simulink model "Adaptive_control_CSAD_model"  (R2017a)
settings: Solver=ode4  StartTime=0.0  StopTime=t_sim  FixedStep=0.01  RelTol=1e-3
values from neighbouring files (symbols this model uses):
  controller = 1    [Run4corner.m]
  eta_initial = [5; -1; 0]    [Run4corner.m]    (also in Simulation_plot.m = [-4; -2; 0.6*pi])
  gamma = 1.5    [Run4corner.m]
  mrs_select = 0    [Run4corner.m]
  nu_initial = [0; 0; 0]    [Run4corner.m]    (also in Simulation_plot.m)
  rho = 0.8    [Run4corner.m]
  sigma = 2    [Run4corner.m]
undefined symbols (not defined in the file or in its folder): fdesignblkfcn, gcbh
libraries: simulink x4, dsparch4 x1
(part 1 of 2)
settings Model: Creator=torees  LastModifiedBy=torees

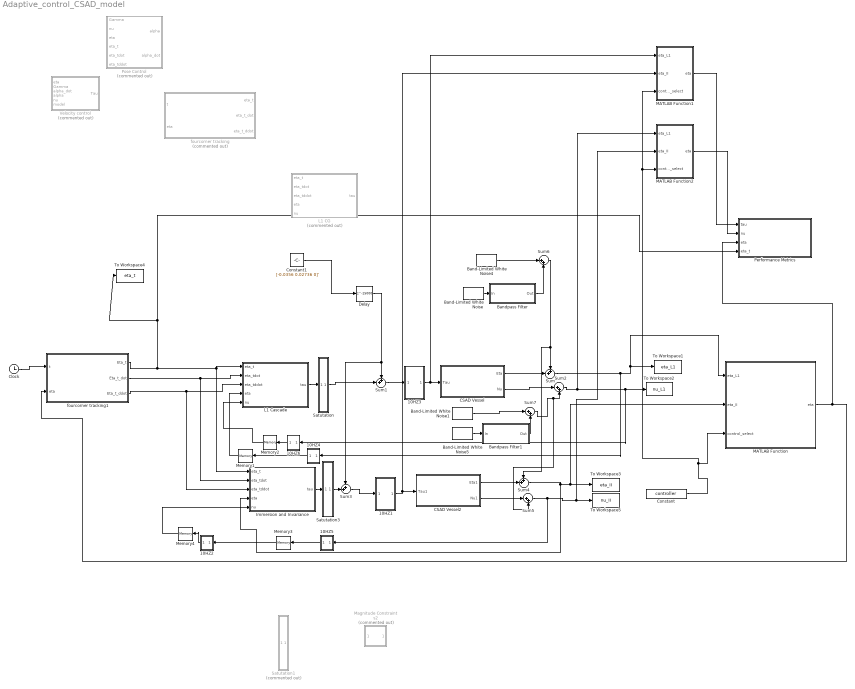
== system Adaptive_control_CSAD_model ==
  10HZ1 : Subsystem
  10HZ2 : Subsystem
  10HZ3 : Subsystem
  10HZ4 : Subsystem
  10HZ5 : Subsystem
  10HZ6 : Subsystem
  Band-Limited White Noise : simulink/Sources/Band-Limited White Noise  Cov=posnoise  Ts=0.01  seed=[233451]
  Band-Limited White Noise1 : simulink/Sources/Band-Limited White Noise  Cov=velnoise2  Ts=0.01  seed=[233451]
  Band-Limited White Noise4 : simulink/Sources/Band-Limited White Noise  Cov=posnoise2  Ts=0.01  seed=[233451]
  Band-Limited White Noise5 : simulink/Sources/Band-Limited White Noise  Cov=velnoise  Ts=0.01  seed=[233451]
  Bandpass Filter : Subsystem  DialogController=fdesignblkfcn  InitFcn=fdesignblkfcn(gcbh, {'InitFcn'});  mask(Bandpass Filter){}
      mask help: Design a bandpass filter
      settings: CopyFcn=fdesignblkfcn(gcbh, {'CopyFcn'});
      mask Help: helpview(mapfilelocation('dsp'), 'dspbandpassfilter');
      mask Display: disp('Bandpass');
  Bandpass Filter1 : Subsystem  DialogController=fdesignblkfcn  InitFcn=fdesignblkfcn(gcbh, {'InitFcn'});  mask(Bandpass Filter){}
      mask help: Design a bandpass filter
      settings: CopyFcn=fdesignblkfcn(gcbh, {'CopyFcn'});
      mask Help: helpview(mapfilelocation('dsp'), 'dspbandpassfilter');
      mask Display: disp('Bandpass');
  CSAD Vessel : Subsystem
  CSAD Vessel2 : Subsystem
  Clock : Clock
  Constant : Constant  Value=controller
  Constant1 : Constant  Value=[-0.0356 0.02736 0]'
  Delay : Delay  DelayLength=15000  InitialCondition=0
  Immersion and Invariance : Subsystem
  L1 CG : Subsystem  Commented=on
  L1 Cascade : Subsystem
  MATLAB Function : MATLAB Function  TreatAsAtomicUnit=on
  MATLAB Function1 : MATLAB Function  TreatAsAtomicUnit=on
  MATLAB Function2 : MATLAB Function  TreatAsAtomicUnit=on
  Magnitude Constraints2 : MATLAB Function  Commented=on  TreatAsAtomicUnit=on
  Memory{1..4} (4 alike) : Memory  X0=[ 0 0 0]'
  "Performance Metrics " : Subsystem
  Pose Control : Subsystem  Commented=on
  Satutation : Subsystem
  Satutation1 : Subsystem  Commented=on
  Satutation3 : Subsystem
  Sum{,1,3..4} (4 alike) : Sum  Inputs=++|
  Sum{2,5..7} (4 alike) : Sum  Inputs=|++
  To Workspace1 : ToWorkspace  VariableName=eta_L1  SampleTime=-1
  To Workspace2 : ToWorkspace  VariableName=nu_L1  SampleTime=-1
  To Workspace3 : ToWorkspace  VariableName=eta_II  SampleTime=-1
  To Workspace4 : ToWorkspace  VariableName=eta_t  SampleTime=-1
  To Workspace5 : ToWorkspace  VariableName=nu_II  SampleTime=-1
  Velocity control : Subsystem  Commented=on
  fourcorner tracking : Subsystem  Commented=on
  fourcorner tracking1 : MATLAB Function  TreatAsAtomicUnit=on
  wires:
  Clock/1 -> fourcorner tracking1/1(t)
  Constant/1 -> MATLAB Function2/3(control_select), MATLAB Function1/3(control_select), MATLAB Function/3(control_select)
  MATLAB Function/1(eta) -> "Performance Metrics "/3(eta), fourcorner tracking1/2(eta)
  CSAD Vessel/1(Eta) -> Sum/2
  fourcorner tracking1/2(Eta_t_dot) -> L1 Cascade/2(eta_tdot), Immersion and Invariance/2(eta_tdot)
  fourcorner tracking1/3(Eta_t_ddot) -> L1 Cascade/3(eta_tddot), Immersion and Invariance/3(eta_tddot)
  Band-Limited White Noise/1 -> Bandpass Filter/1(In)
  10HZ3/1(Out1) -> MATLAB Function1/1(eta_L1), CSAD Vessel/1(Tau)
  Sum/1 -> 10HZ4/1(In1), MATLAB Function/1(eta_L1), To Workspace1/1
  fourcorner tracking1/1(Eta_t) -> To Workspace4/1, "Performance Metrics "/4(eta_t), L1 Cascade/1(eta_t), Immersion and Invariance/1(eta_t)
  L1 Cascade/1(tau) -> Satutation/1(In1)
  Sum1/1 -> 10HZ3/1(In1)
  CSAD Vessel/2(Nu) -> Sum2/1
  Sum7/1 -> Sum5/2, Sum2/2
  Sum2/1 -> MATLAB Function2/1(eta_L1), 10HZ6/1(In1), To Workspace2/1
  Delay/1 -> Sum3/1, Sum1/1
  Immersion and Invariance/1(tau) -> Satutation3/1(In1)
  Sum3/1 -> 10HZ1/1(In1)
  CSAD Vessel2/1(Eta1) -> Sum4/2
  CSAD Vessel2/2(Nu1) -> Sum5/1
  Sum5/1 -> 10HZ5/1(In1), MATLAB Function2/2(eta_II), To Workspace5/1
  Sum4/1 -> Immersion and Invariance/4(eta), MATLAB Function/2(eta_II), To Workspace3/1
  10HZ1/1(Out1) -> CSAD Vessel2/1(Tau1), MATLAB Function1/2(eta_II)
  MATLAB Function1/1(eta) -> "Performance Metrics "/1(tau)
  MATLAB Function2/1(eta) -> "Performance Metrics "/2(nu)
  Satutation/1(Out1) -> Sum1/2
  Satutation3/1(Out1) -> Sum3/2
  Bandpass Filter/1(Out) -> Sum6/2
  Sum6/1 -> Sum4/1, Sum/1
  Band-Limited White Noise4/1 -> Sum6/1
  Bandpass Filter1/1(Out) -> Sum7/2
  Band-Limited White Noise5/1 -> Bandpass Filter1/1(In)
  Band-Limited White Noise1/1 -> Sum7/1
  Constant1/1 -> Delay/1
  10HZ2/1(Out1) -> Memory4/1
  10HZ5/1(Out1) -> Memory3/1
  Memory3/1 -> 10HZ2/1(In1)
  Memory4/1 -> Immersion and Invariance/5(nu)
  Memory1/1 -> L1 Cascade/4(eta)
  Memory2/1 -> L1 Cascade/5(nu)
  10HZ6/1(Out1) -> Memory2/1
  10HZ4/1(Out1) -> Memory1/1

== system Adaptive_control_CSAD_model/10HZ1 ==
  In1 : Inport
  MATLAB Function : MATLAB Function  TreatAsAtomicUnit=on
  Memory : Memory
  Memory1 : Memory
  Out1 : Outport
  wires:
  In1/1 -> MATLAB Function/1(nu)
  MATLAB Function/1(nu_10) -> Memory1/1, Out1/1
  Memory1/1 -> MATLAB Function/2(nu_current)
  MATLAB Function/2(i_out) -> Memory/1
  Memory/1 -> MATLAB Function/3(i)

== system Adaptive_control_CSAD_model/10HZ2 ==
  In1 : Inport
  MATLAB Function : MATLAB Function  TreatAsAtomicUnit=on
  Memory : Memory
  Memory1 : Memory
  Out1 : Outport
  wires:
  In1/1 -> MATLAB Function/1(nu)
  MATLAB Function/1(nu_10) -> Memory1/1, Out1/1
  Memory1/1 -> MATLAB Function/2(nu_current)
  MATLAB Function/2(i_out) -> Memory/1
  Memory/1 -> MATLAB Function/3(i)

== system Adaptive_control_CSAD_model/10HZ3 ==
  In1 : Inport
  MATLAB Function : MATLAB Function  TreatAsAtomicUnit=on
  Memory : Memory
  Memory1 : Memory
  Out1 : Outport
  wires:
  In1/1 -> MATLAB Function/1(nu)
  MATLAB Function/1(nu_10) -> Memory1/1, Out1/1
  Memory1/1 -> MATLAB Function/2(nu_current)
  MATLAB Function/2(i_out) -> Memory/1
  Memory/1 -> MATLAB Function/3(i)

== system Adaptive_control_CSAD_model/10HZ4 ==
  In1 : Inport
  MATLAB Function : MATLAB Function  TreatAsAtomicUnit=on
  Memory : Memory
  Memory1 : Memory
  Out1 : Outport
  wires:
  In1/1 -> MATLAB Function/1(nu)
  MATLAB Function/1(nu_10) -> Memory1/1, Out1/1
  Memory1/1 -> MATLAB Function/2(nu_current)
  MATLAB Function/2(i_out) -> Memory/1
  Memory/1 -> MATLAB Function/3(i)

== system Adaptive_control_CSAD_model/10HZ5 ==
  In1 : Inport
  MATLAB Function : MATLAB Function  TreatAsAtomicUnit=on
  Memory : Memory
  Memory1 : Memory
  Out1 : Outport
  wires:
  In1/1 -> MATLAB Function/1(nu)
  MATLAB Function/1(nu_10) -> Memory1/1, Out1/1
  Memory1/1 -> MATLAB Function/2(nu_current)
  MATLAB Function/2(i_out) -> Memory/1
  Memory/1 -> MATLAB Function/3(i)

== system Adaptive_control_CSAD_model/10HZ6 ==
  In1 : Inport
  MATLAB Function : MATLAB Function  TreatAsAtomicUnit=on
  Memory : Memory
  Memory1 : Memory
  Out1 : Outport
  wires:
  In1/1 -> MATLAB Function/1(nu)
  MATLAB Function/1(nu_10) -> Memory1/1, Out1/1
  Memory1/1 -> MATLAB Function/2(nu_current)
  MATLAB Function/2(i_out) -> Memory/1
  Memory/1 -> MATLAB Function/3(i)

== system Adaptive_control_CSAD_model/Bandpass Filter ==
  In : Inport
  Generated Filter Block : dsparch4/Biquad Filter  Tag=BlockMethodSubSystem  IIRFiltStruct=Direct form II  CoeffSource=Specify via dialog  BiQuadCoeffs=[0.28932621448050977 -0.19800857833013893 0.28932621448050977 1 -0.62679229449728924 0.99326477861490148;2 -1.1003519967587603 2 1 -0.60508947521969358 0.99323977127646146]  a0Flag=Warning  IC=0  ICnum=0  ICden=0  denAccumFracLength=30  denProdOutputFracLength=30  secondMemoryFracLength=15  roundingMode=Floor  overflowMode=off  ScaleValues=[0.0063942944592789474;1;8.4992509081585865]  optimizeScaleValues=off  ScaleValueMode=Specify via input port (g)  scaleValueFracLength=14  FilterSource=Specify via dialog  FilterObject=BQF
      settings: SourceProductName=DSP System Toolbox
  Out : Outport
  wires:
  In/1 -> Generated Filter Block/1
  Generated Filter Block/1 -> Out/1

== system Adaptive_control_CSAD_model/Bandpass Filter1 ==
  In : Inport
  Generated Filter Block : DiscreteFir  Tag=BlockMethodSubSystem  Coefficients=[-0.00022866080475683346 9.0500149570757829e-05 0.00030323221623319483 9.6950387506687544e-05 -0.00026242642230850892 -0.0002711366425355462 0.00010692965569039904 0.00035703592389110518 0.0001137646206031183 -0.00030691485656133589 -0.00031606842611407629 0.00012425156584503172 0.00041357392060654058 0.00013137455407803862 -0.00035335288906473983 -0.00036281158309483126 0.00014221078759315593 0.00047199197512735132 0.00014950735046501945 -0.0004010030641912538 -0.00041060556794784119 0.00016050803082857278 0.00053129325037747273 0.00016784626486823976 -0.00044901347408479709 -0.00045857596188389704 0.00017880076164063021 0.00059034188467914416 0.0001860319053437639 -0.00049642146300410558 -0.00050573858373898569 0.00019670492845249974 0.00064786908395723572 0.00020366427238696581 -0.00054215937839953313 -0.00055100565329149829 0.0002137974737911931 0.00070248176006464037 0.00022030558586361808 -0.00058506238388481176 -0.00059319401544844787 0.00022961963232185327 0.00075267370883052502 0.00023548389477967926 -0.00062387831512850491 -0.00063103539936720581 0.00024368100257043411 0.00079683927845801926 0.00024869745194265759 -0.00065727952461614076 -0.00066318865138829323 0.00025546436628043524 0.00083328943519669484 0.00025941982204517541 -0.00068387662581250168 -0.00068825384523529679 0.00026443121583222024 0.00086027008953348458 0.00026710567823234714 -0.00070223401209240611 -0.00070478813790462915 0.00027002793682867539 0.00087598250324764709 0.00027119722903582057 -0.00071088699153184977 -0.0007113232056427276 0.0002716925800607281 0.00087860555633217539 0.00027113120490539699 -0.00070836034588075394 -0.00070638406201184434 0.00026886214484442235 0.00086631961375804867 0.00026634632168098132 -0.00069318809138455863 -0.00068850902988833445 0.00026098028439975311 0.00083733169609006826 0.00025629112744891548 -0.00066393419117570518 -0.00065627061189895536 0.00024750533374148212 0.00078990162576007068 0.00024043212953145016 -0.00061921394427171374 -0.00060829697983306812 0.00022791855167660663 0.00072236879301993025 0.00021826209007098061 -0.00055771575530826458 -0.00054329378347130338 0.00020173246114520867 0.00063317916282721166 0.00018930837196203979 -0.00047822297245887248 -0.00046006596349108212 0.00016849916646111482 0.00052091212668398058 0.00015314121191948102 -0.00037963546894463184 -0.00035753924202824091 0.00012781852215017049 0.0003843067921841167 0.0001093817943726065 -0.00026099063643892322 -0.00023478095839591449 7.9346026156598272e-05 0.00022228729807382744 5.7709998744626233e-05 -0.0001214834567673515 -9.1019916619938159e-05 2.2800310273292612e-05 3.3986744229492286e-05 -2.128306417296879e-06 3.9514678247534553e-05 7.4335084020332669e-05 -4.202989720410375e-05 -0.00018123066576116855 -7.0314546022854377e-05 0.00022243872007539367 0.00026167835429942682 -0.0001152794573813064 -0.00042374965674570259 -0.00014695141624931636 0.00042751459690613518 0.00047119235971186478 -0.00019700126974396431 -0.00069368645462418769 -0.00023205766902919368 0.00065474601466195004 0.00070283498741295538 -0.00028716159046765152 -0.0009908742371996836 -0.00032556380563102225 0.00090390368840259497 0.00095632929273069755 -0.00038563631616019754 -0.0013148517669741538 -0.00042730877086712756 0.0011745172375142614 0.0012311559522155734 -0.00049220831721037879 -0.0016648554699201688 -0.00053703772687117694 0.0014658699442639297 0.0015265486155602746 -0.00060656589137952281 -0.0020398151794789807 -0.00065440097125783704 0.0017769965375642577 0.0018414923102623507 -0.0007283023933155274 -0.0024383537157949228 -0.0007789540490108711 0.002106684122673889 0.0021747250111771332 -0.00085691707950865195 -0.0028587904172171124 -0.0009101590908727656 0.0024534763336618096 0.0025247424427352594 -0.00099181719108769242 -0.0032991486851696498 -0.0010473873935739611 0.0028156807394573154 0.0028898061352528822 -0.0011323212790349943 -0.0037571675454802682 -0.001189923239218751 0.0031913794869021191 0.0032679547091675597 -0.0012776637581563624 ...(+8838 chars)]  InputProcessing=Columns as channels (frame based)
  Out : Outport
  wires:
  In/1 -> Generated Filter Block/1
  Generated Filter Block/1 -> Out/1

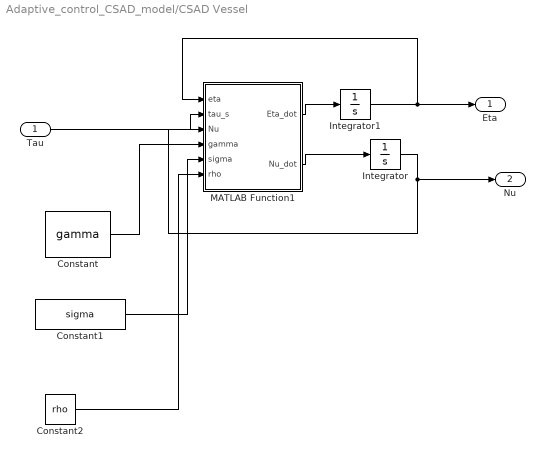
== system Adaptive_control_CSAD_model/CSAD Vessel ==
  Tau : Inport
  Constant : Constant  Value=gamma
  Constant1 : Constant  Value=sigma
  Constant2 : Constant  Value=rho
  Integrator : Integrator  InitialCondition=nu_initial
  Integrator1 : Integrator  InitialCondition=eta_initial
  MATLAB Function1 : MATLAB Function  TreatAsAtomicUnit=on
  Eta : Outport
  Nu : Outport  Port=2
  wires:
  Integrator/1 -> Nu/1, MATLAB Function1/3(Nu)
  MATLAB Function1/1(Eta_dot) -> Integrator1/1
  Integrator1/1 -> Eta/1, MATLAB Function1/1(eta)
  MATLAB Function1/2(Nu_dot) -> Integrator/1
  Tau/1 -> MATLAB Function1/2(tau_s)
  Constant/1 -> MATLAB Function1/4(gamma)
  Constant1/1 -> MATLAB Function1/5(sigma)
  Constant2/1 -> MATLAB Function1/6(rho)

== system Adaptive_control_CSAD_model/CSAD Vessel2 ==
  Tau1 : Inport
  Constant2 : Constant  Value=gamma
  Constant3 : Constant  Value=sigma
  Constant4 : Constant  Value=rho
  Integrator2 : Integrator  InitialCondition=nu_initial
  Integrator3 : Integrator  InitialCondition=eta_initial
  MATLAB Function2 : MATLAB Function  TreatAsAtomicUnit=on
  Eta1 : Outport
  Nu1 : Outport  Port=2
  wires:
  Constant4/1 -> MATLAB Function2/6(rho)
  MATLAB Function2/2(Nu_dot) -> Integrator2/1
  Tau1/1 -> MATLAB Function2/2(tau_s)
  Integrator3/1 -> Eta1/1, MATLAB Function2/1(eta)
  Constant2/1 -> MATLAB Function2/4(gamma)
  MATLAB Function2/1(Eta_dot) -> Integrator3/1
  Constant3/1 -> MATLAB Function2/5(sigma)
  Integrator2/1 -> Nu1/1, MATLAB Function2/3(Nu)

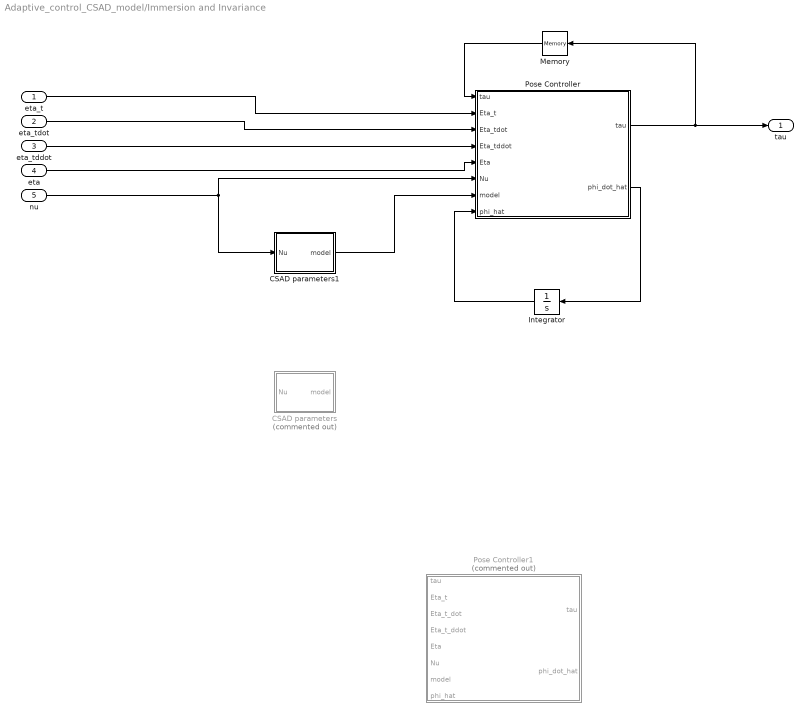
== system Adaptive_control_CSAD_model/Immersion and Invariance ==
  eta_t : Inport
  eta_tdot : Inport  Port=2
  eta_tddot : Inport  Port=3
  eta : Inport  Port=4
  nu : Inport  Port=5
  " Pose Controller" : MATLAB Function  TreatAsAtomicUnit=on
  " Pose Controller1" : MATLAB Function  Commented=on  TreatAsAtomicUnit=on
  CSAD parameters : MATLAB Function  Commented=on  TreatAsAtomicUnit=on
  CSAD parameters1 : MATLAB Function  TreatAsAtomicUnit=on
  Integrator : Integrator
  Memory : Memory  X0=[0 0 0]'
  tau : Outport
  wires:
  eta/1 -> " Pose Controller"/5(Eta)
  nu/1 -> CSAD parameters1/1(Nu), " Pose Controller"/6(Nu)
  " Pose Controller"/1(tau) -> Memory/1, tau/1
  Memory/1 -> " Pose Controller"/1("tau ")
  eta_t/1 -> " Pose Controller"/2(Eta_t)
  eta_tdot/1 -> " Pose Controller"/3(Eta_tdot)
  eta_tddot/1 -> " Pose Controller"/4(Eta_tddot)
  CSAD parameters1/1(model) -> " Pose Controller"/7(model)
  Integrator/1 -> " Pose Controller"/8(phi_hat)
  " Pose Controller"/2(phi_dot_hat) -> Integrator/1

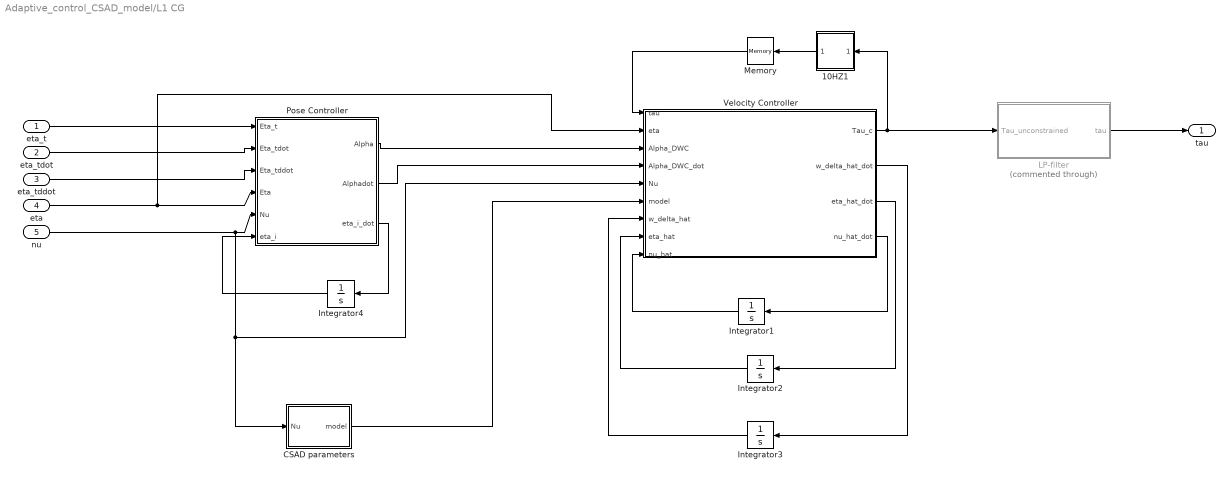
== system Adaptive_control_CSAD_model/L1 CG ==
  eta_t : Inport
  eta_tdot : Inport  Port=2
  eta_tddot : Inport  Port=3
  eta : Inport  Port=4
  nu : Inport  Port=5
  " Pose Controller" : MATLAB Function  TreatAsAtomicUnit=on
  " Velocity Controller" : MATLAB Function  TreatAsAtomicUnit=on
  10HZ1 : Subsystem
  CSAD parameters : MATLAB Function  TreatAsAtomicUnit=on
  Integrator1 : Integrator
  Integrator2 : Integrator
  Integrator3 : Integrator
  Integrator4 : Integrator  InitialCondition=[0 0 0]'
  LP-filter : Subsystem  Commented=through
  Memory : Memory  X0=[0 0 0]'
  tau : Outport
  wires:
  eta_t/1 -> " Pose Controller"/1(Eta_t)
  Memory/1 -> " Velocity Controller"/1(tau)
  " Velocity Controller"/1(Tau_c) -> LP-filter/1(Tau_unconstrained), 10HZ1/1(In1)
  " Velocity Controller"/4(nu_hat_dot) -> Integrator1/1
  Integrator1/1 -> " Velocity Controller"/9(nu_hat)
  " Velocity Controller"/3(eta_hat_dot) -> Integrator2/1
  Integrator2/1 -> " Velocity Controller"/8(eta_hat)
  " Velocity Controller"/2(w_delta_hat_dot) -> Integrator3/1
  Integrator3/1 -> " Velocity Controller"/7(w_delta_hat)
  eta_tdot/1 -> " Pose Controller"/2(Eta_tdot)
  eta_tddot/1 -> " Pose Controller"/3(Eta_tddot)
  eta/1 -> " Velocity Controller"/2(eta), " Pose Controller"/4(Eta)
  nu/1 -> " Velocity Controller"/5(Nu), CSAD parameters/1(Nu), " Pose Controller"/5(Nu)
  CSAD parameters/1(model) -> " Velocity Controller"/6(model)
  " Pose Controller"/2(Alphadot) -> " Velocity Controller"/4(Alpha_DWC_dot)
  " Pose Controller"/1(Alpha) -> " Velocity Controller"/3(Alpha_DWC)
  LP-filter/1(tau) -> tau/1
  " Pose Controller"/3(eta_i_dot) -> Integrator4/1
  Integrator4/1 -> " Pose Controller"/6(eta_i)
  10HZ1/1(Out1) -> Memory/1

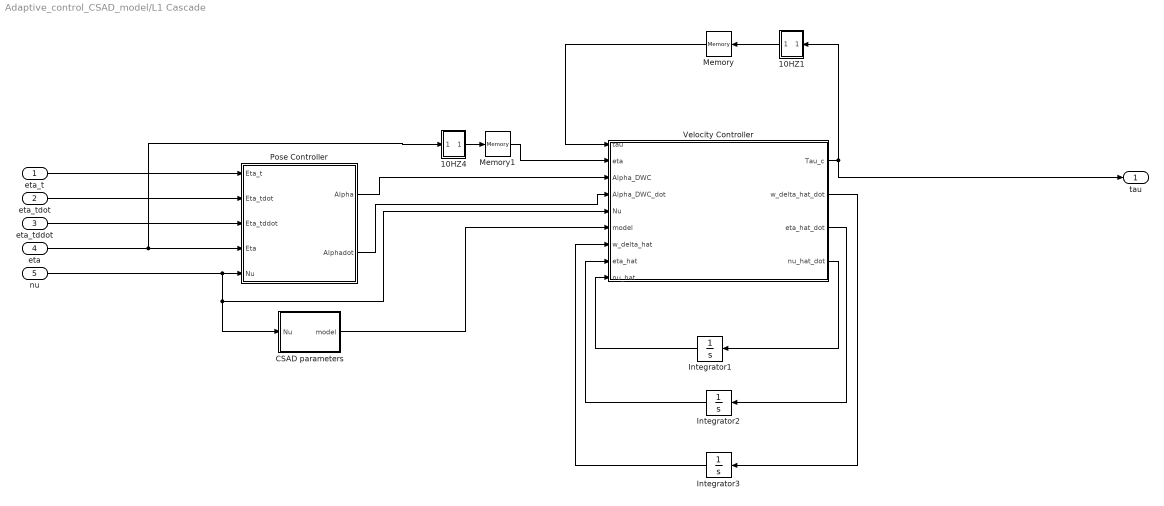
== system Adaptive_control_CSAD_model/L1 Cascade ==
  eta_t : Inport
  eta_tdot : Inport  Port=2
  eta_tddot : Inport  Port=3
  eta : Inport  Port=4
  nu : Inport  Port=5
  " Pose Controller" : MATLAB Function  TreatAsAtomicUnit=on
  10HZ1 : Subsystem
  10HZ4 : Subsystem
  CSAD parameters : MATLAB Function  TreatAsAtomicUnit=on
  Integrator1 : Integrator
  Integrator2 : Integrator  InitialCondition=eta_initial
  Integrator3 : Integrator
  Memory : Memory  X0=[0 0 0]'
  Memory1 : Memory  X0=[ 0 0 0]'
  Velocity Controller : MATLAB Function  TreatAsAtomicUnit=on
  tau : Outport
  wires:
  eta_t/1 -> " Pose Controller"/1(Eta_t)
  Memory/1 -> Velocity Controller/1(tau)
  Velocity Controller/4(nu_hat_dot) -> Integrator1/1
  Integrator1/1 -> Velocity Controller/9(nu_hat)
  Velocity Controller/3(eta_hat_dot) -> Integrator2/1
  Integrator2/1 -> Velocity Controller/8(eta_hat)
  Velocity Controller/2(w_delta_hat_dot) -> Integrator3/1
  Integrator3/1 -> Velocity Controller/7(w_delta_hat)
  eta_tdot/1 -> " Pose Controller"/2(Eta_tdot)
  eta_tddot/1 -> " Pose Controller"/3(Eta_tddot)
  eta/1 -> 10HZ4/1(In1), " Pose Controller"/4(Eta)
  nu/1 -> Velocity Controller/5(Nu), CSAD parameters/1(Nu), " Pose Controller"/5(Nu)
  CSAD parameters/1(model) -> Velocity Controller/6(model)
  " Pose Controller"/2(Alphadot) -> Velocity Controller/4(Alpha_DWC_dot)
  " Pose Controller"/1(Alpha) -> Velocity Controller/3(Alpha_DWC)
  Velocity Controller/1(Tau_c) -> tau/1, 10HZ1/1(In1)
  10HZ4/1(Out1) -> Memory1/1
  Memory1/1 -> Velocity Controller/2(eta)
  10HZ1/1(Out1) -> Memory/1

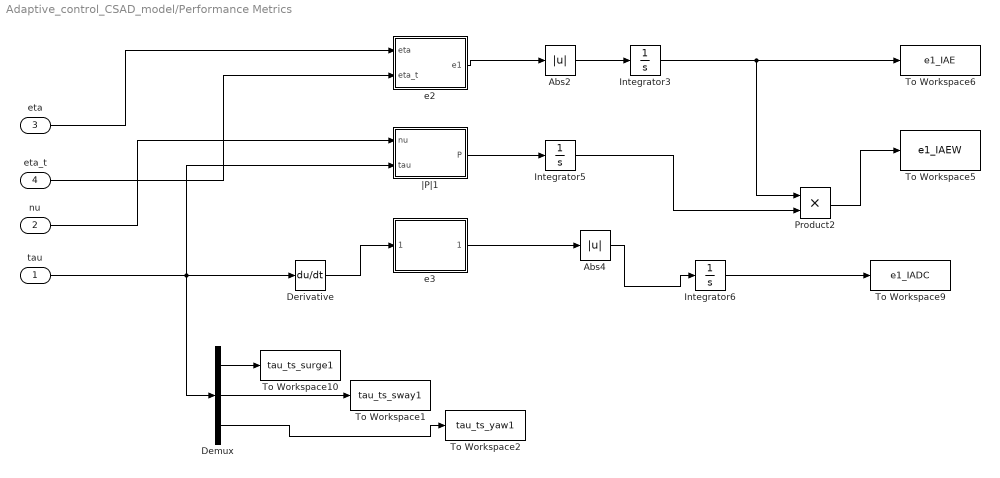
== system Adaptive_control_CSAD_model/Performance Metrics  ==
  tau : Inport
  nu : Inport  Port=2
  eta : Inport  Port=3
  eta_t : Inport  Port=4
  Abs2 : Abs
  Abs4 : Abs
  Demux : Demux  Outputs=3
  Derivative : Derivative
  Integrator3 : Integrator
  Integrator5 : Integrator
  Integrator6 : Integrator
  Product2 : Product
  To Workspace1 : ToWorkspace  VariableName=tau_ts_sway1  SaveFormat=Timeseries  SampleTime=-1
  To Workspace10 : ToWorkspace  VariableName=tau_ts_surge1  SaveFormat=Timeseries  SampleTime=-1
  To Workspace2 : ToWorkspace  VariableName=tau_ts_yaw1  SaveFormat=Timeseries  SampleTime=-1
  To Workspace5 : ToWorkspace  VariableName=e1_IAEW  SaveFormat=Timeseries  SampleTime=-1
  To Workspace6 : ToWorkspace  VariableName=e1_IAE  SaveFormat=Timeseries  SampleTime=-1
  To Workspace9 : ToWorkspace  VariableName=e1_IADC  SaveFormat=Timeseries  SampleTime=-1
  e2 : MATLAB Function  TreatAsAtomicUnit=on
  e3 : MATLAB Function  TreatAsAtomicUnit=on
  |P|1 : MATLAB Function  TreatAsAtomicUnit=on
  wires:
  eta_t/1 -> e2/2(eta_t)
  eta/1 -> e2/1(eta)
  nu/1 -> |P|1/1(nu)
  tau/1 -> |P|1/2(tau), Demux/1, Derivative/1
  Integrator3/1 -> Product2/1, To Workspace6/1
  |P|1/1(P) -> Integrator5/1
  e2/1(e1) -> Abs2/1
  e3/1(tau_dot) -> Abs4/1
  Abs2/1 -> Integrator3/1
  Derivative/1 -> e3/1(tau_dot_in)
  Integrator6/1 -> To Workspace9/1
  Integrator5/1 -> Product2/2
  Product2/1 -> To Workspace5/1
  Abs4/1 -> Integrator6/1
  Demux/1 -> To Workspace10/1
  Demux/2 -> To Workspace1/1
  Demux/3 -> To Workspace2/1

== system Adaptive_control_CSAD_model/Pose Control ==
  Gamma : Inport
  nu : Inport  Port=2
  eta : Inport  Port=3
  eta_t : Inport  Port=4
  eta_tdot : Inport  Port=5
  eta_tddot : Inport  Port=6
  Pose : MATLAB Function  TreatAsAtomicUnit=on
  alpha : Outport
  alpha_dot : Outport  Port=2
  wires:
  Pose/1(alpha) -> alpha/1
  Pose/2(alpha_dot) -> alpha_dot/1
  eta/1 -> Pose/6(eta)
  eta_tdot/1 -> Pose/4(eta_t_dot)
  eta_tddot/1 -> Pose/5(eta_t_ddot)
  eta_t/1 -> Pose/2(eta_t)
  nu/1 -> Pose/3(nu)
  Gamma/1 -> Pose/1(Gamma1)

== system Adaptive_control_CSAD_model/Satutation ==
  In1 : Inport
  Constant : Constant  Value=mrs_select
  MATLAB Function1 : MATLAB Function  TreatAsAtomicUnit=on
  MRS 2 : Subsystem
  Out1 : Outport
  wires:
  In1/1 -> MRS 2/1(Tau_c), MATLAB Function1/1(tau)
  MRS 2/1(Tau_mrs) -> MATLAB Function1/2(tau_mrs)
  MATLAB Function1/1(tau_out) -> Out1/1
  Constant/1 -> MATLAB Function1/3(mrs)

== system Adaptive_control_CSAD_model/Satutation1 ==
  In1 : Inport
  Constant : Constant  Value=mrs_select
  MATLAB Function1 : MATLAB Function  TreatAsAtomicUnit=on
  MRS 1 : Subsystem
  Out1 : Outport
  wires:
  In1/1 -> MRS 1/1(Tau_c), MATLAB Function1/1(tau)
  MRS 1/1(Tau_mrs) -> MATLAB Function1/2(tau_mrs)
  MATLAB Function1/1(tau_out) -> Out1/1
  Constant/1 -> MATLAB Function1/3(mrs)

== system Adaptive_control_CSAD_model/Satutation3 ==
  In1 : Inport
  Constant : Constant  Value=mrs_select
  MATLAB Function1 : MATLAB Function  TreatAsAtomicUnit=on
  MRS 2 : Subsystem
  Out1 : Outport
  wires:
  In1/1 -> MRS 2/1(Tau_c), MATLAB Function1/1(tau)
  MRS 2/1(Tau_mrs) -> MATLAB Function1/2(tau_mrs)
  MATLAB Function1/1(tau_out) -> Out1/1
  Constant/1 -> MATLAB Function1/3(mrs)

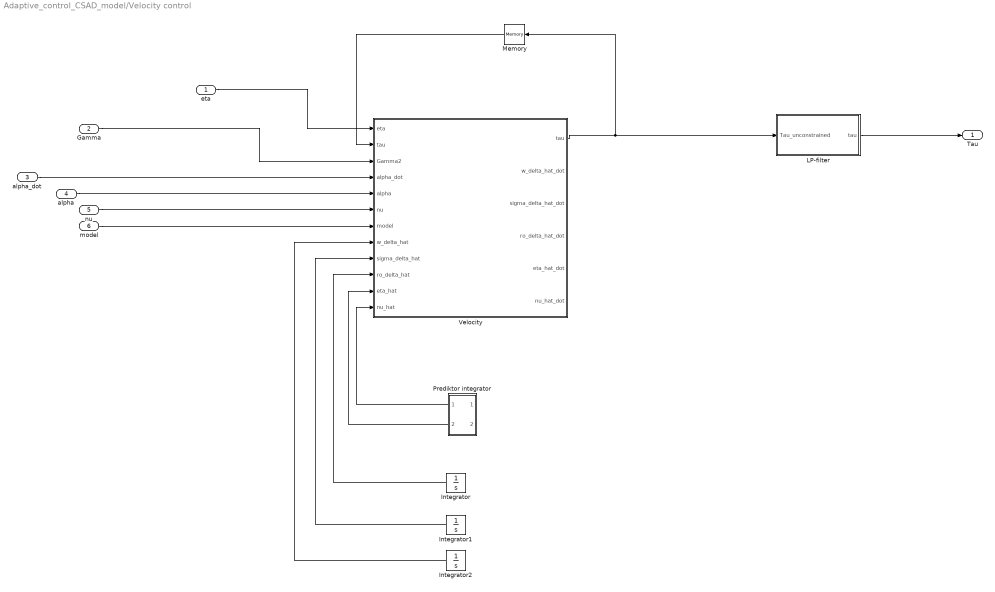
== system Adaptive_control_CSAD_model/Velocity control ==
  eta : Inport
  Gamma : Inport  Port=2
  alpha_dot : Inport  Port=3
  alpha : Inport  Port=4
  nu : Inport  Port=5
  model : Inport  Port=6
  Integrator : Integrator  InitialCondition=1
  Integrator1 : Integrator  InitialCondition=1
  Integrator2 : Integrator  InitialCondition=[0, 0, 0]'
  LP-filter : Subsystem
  Memory : Memory  X0=[0 0 0]
  Prediktor integrator : Subsystem
  Velocity : MATLAB Function  TreatAsAtomicUnit=on
  Tau : Outport
  wires:
  alpha_dot/1 -> Velocity/4(alpha_dot)
  alpha/1 -> Velocity/5(alpha)
  nu/1 -> Velocity/6(nu)
  Velocity/1(tau) -> LP-filter/1(Tau_unconstrained), Memory/1
  model/1 -> Velocity/7(model)
  Gamma/1 -> Velocity/3(Gamma2)
  Prediktor integrator/1(Out2) -> Velocity/12(nu_hat)
  Integrator1/1 -> Velocity/9(sigma_delta_hat)
  Integrator2/1 -> Velocity/8(w_delta_hat)
  Prediktor integrator/2(Out1) -> Velocity/11(eta_hat)
  Integrator/1 -> Velocity/10(ro_delta_hat)
  Memory/1 -> Velocity/2("tau ")
  LP-filter/1(tau) -> Tau/1
  eta/1 -> Velocity/1(eta)

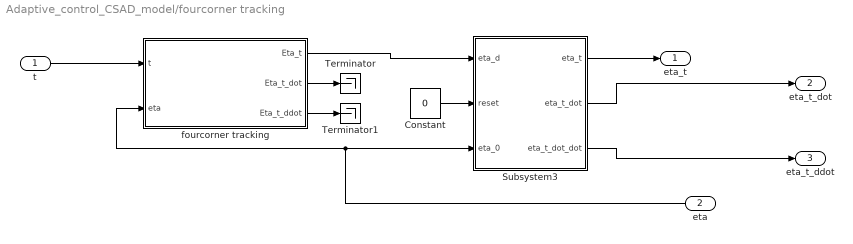
== system Adaptive_control_CSAD_model/fourcorner tracking ==
  t : Inport
  eta : Inport  Port=2
  Constant : Constant  Value=0
  Subsystem3 : Subsystem
  Terminator : Terminator
  Terminator1 : Terminator
  fourcorner tracking : MATLAB Function  TreatAsAtomicUnit=on
  eta_t : Outport
  eta_t_dot : Outport  Port=2
  eta_t_ddot : Outport  Port=3
  wires:
  Subsystem3/3(eta_t_dot_dot) -> eta_t_ddot/1
  fourcorner tracking/2(Eta_t_dot) -> Terminator/1
  Constant/1 -> Subsystem3/2(reset)
  Subsystem3/1(eta_t) -> eta_t/1
  t/1 -> fourcorner tracking/1(t)
  eta/1 -> fourcorner tracking/2(eta), Subsystem3/3(eta_0)
  fourcorner tracking/3(Eta_t_ddot) -> Terminator1/1
  fourcorner tracking/1(Eta_t) -> Subsystem3/1(eta_d)
  Subsystem3/2(eta_t_dot) -> eta_t_dot/1

== system Adaptive_control_CSAD_model/L1 CG/10HZ1 ==
  In1 : Inport
  MATLAB Function : MATLAB Function  TreatAsAtomicUnit=on
  Memory : Memory
  Memory1 : Memory
  Out1 : Outport
  wires:
  In1/1 -> MATLAB Function/1(nu)
  MATLAB Function/1(nu_10) -> Memory1/1, Out1/1
  Memory1/1 -> MATLAB Function/2(nu_current)
  MATLAB Function/2(i_out) -> Memory/1
  Memory/1 -> MATLAB Function/3(i)

== system Adaptive_control_CSAD_model/L1 CG/LP-filter ==
  Tau_unconstrained : Inport
  Demux : Demux  Outputs=3
  Mux : Mux  Inputs=3
  Transfer Fcn1 : TransferFcn  Numerator=[100]  Denominator=[1 100]
  Transfer Fcn2 : TransferFcn  Numerator=[100]  Denominator=[1 100]
  Transfer Fcn3 : TransferFcn  Numerator=[100]  Denominator=[1 100]
  tau : Outport
  wires:
  Transfer Fcn1/1 -> Mux/1
  Demux/2 -> Transfer Fcn3/1
  Mux/1 -> tau/1
  Demux/1 -> Transfer Fcn1/1
  Transfer Fcn2/1 -> Mux/3
  Transfer Fcn3/1 -> Mux/2
  Demux/3 -> Transfer Fcn2/1
  Tau_unconstrained/1 -> Demux/1

== system Adaptive_control_CSAD_model/L1 Cascade/10HZ1 ==
  In1 : Inport
  MATLAB Function : MATLAB Function  TreatAsAtomicUnit=on
  Memory : Memory
  Memory1 : Memory
  Out1 : Outport
  wires:
  In1/1 -> MATLAB Function/1(nu)
  MATLAB Function/1(nu_10) -> Memory1/1, Out1/1
  Memory1/1 -> MATLAB Function/2(nu_current)
  MATLAB Function/2(i_out) -> Memory/1
  Memory/1 -> MATLAB Function/3(i)

== system Adaptive_control_CSAD_model/L1 Cascade/10HZ4 ==
  In1 : Inport
  MATLAB Function : MATLAB Function  TreatAsAtomicUnit=on
  Memory : Memory
  Memory1 : Memory
  Out1 : Outport
  wires:
  In1/1 -> MATLAB Function/1(nu)
  MATLAB Function/1(nu_10) -> Memory1/1, Out1/1
  Memory1/1 -> MATLAB Function/2(nu_current)
  MATLAB Function/2(i_out) -> Memory/1
  Memory/1 -> MATLAB Function/3(i)

== system Adaptive_control_CSAD_model/Satutation/MRS 2 ==
  Tau_c : Inport
  Derivative : Derivative
  Gain : Gain  Gain=diag([5,2.78,2.36])  Multiplication=Matrix(K*u)
  Integrator1 : Integrator  InitialCondition=[0;0;0]
  Magnitude Constraints2 : MATLAB Function  TreatAsAtomicUnit=on
  Rate Constraints1 : MATLAB Function  TreatAsAtomicUnit=on
  Sum : Sum  Inputs=++|
  Sum1 : Sum  Inputs=+|-
  Tau_mrs : Outport
  wires:
  Gain/1 -> Sum/1
  Sum1/1 -> Gain/1
  Magnitude Constraints2/1(Tau_mrs) -> Tau_mrs/1
  Integrator1/1 -> Magnitude Constraints2/1(delta), Sum1/2
  Rate Constraints1/1(delta_dot) -> Integrator1/1
  Sum/1 -> Rate Constraints1/1(epsilon)
  Derivative/1 -> Sum/2
  Tau_c/1 -> Derivative/1, Sum1/1

== system Adaptive_control_CSAD_model/Satutation1/MRS 1 ==
  Tau_c : Inport
  Derivative : Derivative
  Gain : Gain  Gain=diag([4;3;2])  Multiplication=Matrix(K*u)
  Integrator1 : Integrator  InitialCondition=[0;0;0]
  Magnitude Constraints2 : MATLAB Function  TreatAsAtomicUnit=on
  Rate Constraints1 : MATLAB Function  TreatAsAtomicUnit=on
  Sum : Sum  Inputs=++|
  Sum1 : Sum  Inputs=+|-
  Tau_mrs : Outport
  wires:
  Gain/1 -> Sum/1
  Sum1/1 -> Gain/1
  Magnitude Constraints2/1(Tau_mrs) -> Tau_mrs/1
  Integrator1/1 -> Magnitude Constraints2/1(delta), Sum1/2
  Rate Constraints1/1(delta_dot) -> Integrator1/1
  Sum/1 -> Rate Constraints1/1(epsilon)
  Derivative/1 -> Sum/2
  Tau_c/1 -> Derivative/1, Sum1/1

== system Adaptive_control_CSAD_model/Satutation3/MRS 2 ==
  Tau_c : Inport
  Derivative : Derivative
  Gain : Gain  Gain=diag([5,2.78,2.36])  Multiplication=Matrix(K*u)
  Integrator1 : Integrator  InitialCondition=[0;0;0]
  Magnitude Constraints2 : MATLAB Function  TreatAsAtomicUnit=on
  Rate Constraints1 : MATLAB Function  TreatAsAtomicUnit=on
  Sum : Sum  Inputs=++|
  Sum1 : Sum  Inputs=+|-
  Tau_mrs : Outport
  wires:
  Gain/1 -> Sum/1
  Sum1/1 -> Gain/1
  Magnitude Constraints2/1(Tau_mrs) -> Tau_mrs/1
  Integrator1/1 -> Magnitude Constraints2/1(delta), Sum1/2
  Rate Constraints1/1(delta_dot) -> Integrator1/1
  Sum/1 -> Rate Constraints1/1(epsilon)
  Derivative/1 -> Sum/2
  Tau_c/1 -> Derivative/1, Sum1/1

== system Adaptive_control_CSAD_model/Velocity control/LP-filter ==
  Tau_unconstrained : Inport
  Demux : Demux  Outputs=3
  Mux : Mux  Inputs=3
  Transfer Fcn1 : TransferFcn  Numerator=[100]  Denominator=[1 100]
  Transfer Fcn2 : TransferFcn  Numerator=[100]  Denominator=[1 100]
  Transfer Fcn3 : TransferFcn  Numerator=[100]  Denominator=[1 100]
  tau : Outport
  wires:
  Transfer Fcn1/1 -> Mux/1
  Demux/2 -> Transfer Fcn3/1
  Mux/1 -> tau/1
  Demux/1 -> Transfer Fcn1/1
  Transfer Fcn2/1 -> Mux/3
  Transfer Fcn3/1 -> Mux/2
  Demux/3 -> Transfer Fcn2/1
  Tau_unconstrained/1 -> Demux/1

== system Adaptive_control_CSAD_model/Velocity control/Prediktor integrator ==
  In2 : Inport
  In1 : Inport  Port=2
  Integrator3 : Integrator  InitialCondition=eta_initial
  Integrator4 : Integrator  InitialCondition=nu_initial
  Out2 : Outport
  Out1 : Outport  Port=2
  wires:
  Integrator3/1 -> Out1/1
  Integrator4/1 -> Out2/1
  In1/1 -> Integrator3/1
  In2/1 -> Integrator4/1

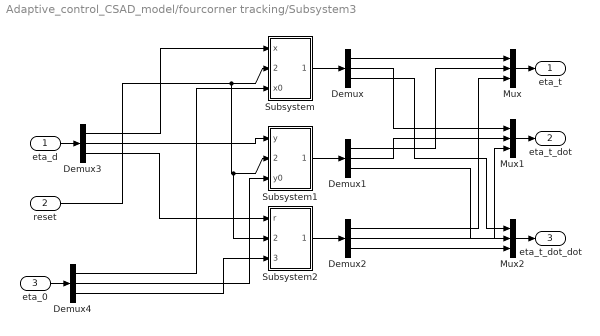
== system Adaptive_control_CSAD_model/fourcorner tracking/Subsystem3 ==
  eta_d : Inport
  reset : Inport  Port=2
  eta_0 : Inport  Port=3
  Demux{,1..4} (5 alike) : Demux  Outputs=3
  Mux : Mux  Inputs=3
  Mux1 : Mux  Inputs=3
  Mux2 : Mux  Inputs=3
  Subsystem : Subsystem
  Subsystem1 : Subsystem
  Subsystem2 : Subsystem
  eta_t : Outport  PortDimensions=3
  eta_t_dot : Outport  Port=2  PortDimensions=3
  eta_t_dot_dot : Outport  Port=3  PortDimensions=3
  wires:
  Subsystem1/1(y,yd,ydd) -> Demux1/1
  Subsystem2/1(y,yd,ydd) -> Demux2/1
  Subsystem/1(x,xd,xdd) -> Demux/1
  Demux/3 -> Mux2/1
  eta_d/1 -> Demux3/1
  Mux1/1 -> eta_t_dot/1
  Demux/1 -> Mux/1
  Mux2/1 -> eta_t_dot_dot/1
  Demux3/1 -> Subsystem/1(x)
  Demux1/3 -> Mux2/2
  Demux2/3 -> Mux2/3
  Demux1/1 -> Mux/2
  Demux3/2 -> Subsystem1/1(y)
  Demux3/3 -> Subsystem2/1(r)
  Demux2/2 -> Mux1/3
  Demux1/2 -> Mux1/2
  reset/1 -> Subsystem2/2(reset), Subsystem1/2(reset), Subsystem/2(reset)
  Mux/1 -> eta_t/1
  Demux/2 -> Mux1/1
  Demux2/1 -> Mux/3
  Demux4/3 -> Subsystem2/3(psi0)
  Demux4/2 -> Subsystem1/3(y0)
  Demux4/1 -> Subsystem/3(x0)
  eta_0/1 -> Demux4/1

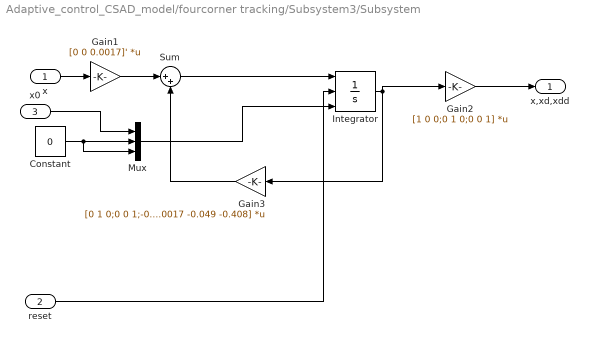
== system Adaptive_control_CSAD_model/fourcorner tracking/Subsystem3/Subsystem ==
  x : Inport
  reset : Inport  Port=2
  x0 : Inport  Port=3
  Constant : Constant  Value=0
  Gain1 : Gain  Gain=[0 0 0.0017]'  Multiplication=Matrix(K*u)
  Gain2 : Gain  Gain=[1 0 0;0 1 0;0 0 1]  Multiplication=Matrix(K*u)
  Gain3 : Gain  Gain=[0 1 0;0 0 1;-0.0017 -0.049 -0.408]  Multiplication=Matrix(K*u)
  Integrator : Integrator  ExternalReset=either  InitialConditionSource=external
  Mux : Mux  Inputs=3
  Sum : Sum  Inputs=|++
  x,xd,xdd : Outport  PortDimensions=3
  wires:
  Gain1/1 -> Sum/1
  x/1 -> Gain1/1
  Integrator/1 -> Gain2/1, Gain3/1
  Sum/1 -> Integrator/1
  Gain2/1 -> x,xd,xdd/1
  Mux/1 -> Integrator/3
  reset/1 -> Integrator/2
  Gain3/1 -> Sum/2
  Constant/1 -> Mux/2, Mux/3
  x0/1 -> Mux/1

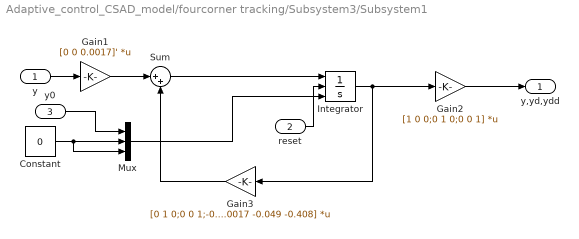
== system Adaptive_control_CSAD_model/fourcorner tracking/Subsystem3/Subsystem1 ==
  y : Inport
  reset : Inport  Port=2
  y0 : Inport  Port=3
  Constant : Constant  Value=0
  Gain1 : Gain  Gain=[0 0 0.0017]'  Multiplication=Matrix(K*u)
  Gain2 : Gain  Gain=[1 0 0;0 1 0;0 0 1]  Multiplication=Matrix(K*u)
  Gain3 : Gain  Gain=[0 1 0;0 0 1;-0.0017 -0.049 -0.408]  Multiplication=Matrix(K*u)
  Integrator : Integrator  ExternalReset=either  InitialConditionSource=external
  Mux : Mux  Inputs=3
  Sum : Sum  Inputs=|++
  y,yd,ydd : Outport
  wires:
  Constant/1 -> Mux/3, Mux/2
  Gain3/1 -> Sum/2
  reset/1 -> Integrator/2
  Mux/1 -> Integrator/3
  Gain2/1 -> y,yd,ydd/1
  Sum/1 -> Integrator/1
  Integrator/1 -> Gain3/1, Gain2/1
  y/1 -> Gain1/1
  Gain1/1 -> Sum/1
  y0/1 -> Mux/1

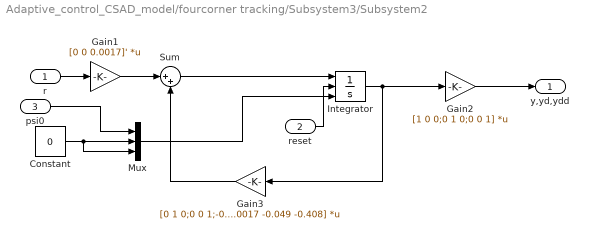
== system Adaptive_control_CSAD_model/fourcorner tracking/Subsystem3/Subsystem2 ==
  r : Inport
  reset : Inport  Port=2
  psi0 : Inport  Port=3
  Constant : Constant  Value=0
  Gain1 : Gain  Gain=[0 0 0.0017]'  Multiplication=Matrix(K*u)
  Gain2 : Gain  Gain=[1 0 0;0 1 0;0 0 1]  Multiplication=Matrix(K*u)
  Gain3 : Gain  Gain=[0 1 0;0 0 1;-0.0017 -0.049 -0.408]  Multiplication=Matrix(K*u)
  Integrator : Integrator  ExternalReset=either  InitialConditionSource=external
  Mux : Mux  Inputs=3
  Sum : Sum  Inputs=|++
  y,yd,ydd : Outport
  wires:
  Gain1/1 -> Sum/1
  r/1 -> Gain1/1
  Integrator/1 -> Gain2/1, Gain3/1
  Sum/1 -> Integrator/1
  Gain2/1 -> y,yd,ydd/1
  Mux/1 -> Integrator/3
  reset/1 -> Integrator/2
  Gain3/1 -> Sum/2
  Constant/1 -> Mux/2, Mux/3
  psi0/1 -> Mux/1

== matlab function Adaptive_control_CSAD_model/Pose Control/Pose ==
  data: Gamma1 input; eta_t input; nu input; eta_t_dot input; eta_t_ddot input; alpha output; alpha_dot output; eta input
function [alpha,alpha_dot]= fcn(Gamma1,eta_t,nu,eta_t_dot,eta_t_ddot,eta)

psi=eta(3);
r=nu(3);
R_T = [cos(psi) -sin(psi) 0;
       sin(psi) cos(psi) 0;
       0 0 1]';
S_T = [0 -r 0;
        r 0 0;
        0 0 0]';

z_1 = R_T*(eta-eta_t);

z1_p_tilde = [z_1(1) z_1(2)]';
z1_psi_tilde = z_1(3);
delta_p_tilde = 0.5;
delta_psi_tilde = 0.5;


K1_func = Gamma1*[ 1/sqrt(z1_p_tilde'*z1_p_tilde + delta_p_tilde^2) 0 0;
                0 1/sqrt(z1_p_tilde'*z1_p_tilde + delta_p_tilde^2) 0;
                0 0 1/sqrt(z1_psi_tilde^2 + delta_psi_tilde^2)];

alpha = R_T*eta_t_dot - K1_func*z_1;            
z_2 = nu-alpha;
z_1_dot = S_T*z_1 - K1_func*z_1 + z_2;
z1_p_tilde_dot = [z_1_dot(1) z_1_dot(2)]';
z1_psi_tilde_dot = z_1_dot(3);
K1_func_dot = -Gamma1*[z1_p_tilde'*z1_p_tilde_dot/((z1_p_tilde'*z1_p_tilde+delta_p_tilde^2)^(3/2)) 0 0;
                0 z1_p_tilde'*z1_p_tilde_dot/((z1_p_tilde'*z1_p_tilde+delta_p_tilde^2)^(3/2)) 0;
                0 0 z1_psi_tilde*z1_psi_tilde_dot/((z1_psi_tilde^2+delta_psi_tilde^2)^(3/2))];

alpha_dot = R_T*eta_t_ddot + S_T*R_T*eta_t_dot - K1_func_dot*z_1 - K1_func*z_1_dot;

== matlab function Adaptive_control_CSAD_model/fourcorner tracking/fourcorner tracking ==
  data: t input; Eta_t output; Eta_t_dot output; Eta_t_ddot output; eta input
function [ Eta_t, Eta_t_dot, Eta_t_ddot]   =  fourcorner_tracking(t,eta)

v_t = 0.15;

etaP = [5 7 7 7 5 5;
       -1 -1 1 1 1 -1;
        0 0 0 pi/4 pi/4 0];
Eta_t_dot = [0;0;0];
Eta_t_ddot = [0;0;0];

Eta_t = [5;-1;0];
persistent point ;
if(isempty(point))
    point = 1;
    
end



switch point
    case 1
        Eta_t = etaP(:,2);
         if ((abs((Eta_t(1)- eta(1))) <0.01 ) ==1  ) && ((abs(Eta_t(2)-eta(2))<0.01) ==1) && (abs(Eta_t(3)-rad2deg(eta(3)))<3 == 1)
            point = 2;
            return;
         end
        
        
    case 2
        Eta_t = etaP(:,3);
        if((abs((Eta_t(1)- eta(1))) <0.01 ) ==1  ) && ((abs(Eta_t(2)-eta(2))<0.01) ==1) && (abs(Eta_t(3)-rad2deg(eta(3)))<3 == 1) 
            point = 3;
            return;
         end
    case 3
        Eta_t = etaP(:,4);
        if((abs((Eta_t(1)- eta(1))) <0.01 ) ==1  ) && ((abs(Eta_t(2)-eta(2))<0.01) ==1) && (rad2deg(abs(Eta_t(3)-eta(3)))<3 == 1)  
            point = 4;
            return;
            
         end
    case 4
        Eta_t = etaP(:,5);
        if((abs((Eta_t(1)- eta(1))) <0.01 ) ==1  ) && ((abs(Eta_t(2)-eta(2))<0.01) ==1) && (rad2deg(abs(Eta_t(3)-eta(3)))<3 == 1) 
            point = 5; 
            return;
         end
    case 5
        Eta_t = etaP(:,6);
        if((abs((Eta_t(1)- eta(1))) <0.01 ) ==1  ) && ((abs(Eta_t(2)-eta(2))<0.01) ==1) && (abs(Eta_t(3)-rad2deg(eta(3)))<3 == 1) 
            point = 6; 
            return;
         end

    otherwise
        

end
end
%(abs(Eta_t(2)-eta(2))<0.01) &&

== matlab function Adaptive_control_CSAD_model/Velocity control/Velocity ==
  data: eta input; tau input; Gamma2 input; alpha_dot input; alpha input; tau output; nu input; model input; w_delta_hat input; sigma_delta_hat input; ro_delta_hat input; eta_hat input; nu_hat input; w_delta_hat_dot output; sigma_delta_hat_dot output; ro_delta_hat_dot output; eta_hat_dot output; nu_hat_dot output
function [tau,w_delta_hat_dot,sigma_delta_hat_dot,ro_delta_hat_dot,eta_hat_dot,nu_hat_dot]= fcn(eta,tau,Gamma2,alpha_dot,alpha,nu,model,w_delta_hat,sigma_delta_hat,ro_delta_hat,eta_hat,nu_hat)
z2=nu-alpha;

M = model(1:3,1:3);
C = model(1:3,4:6);
D = model(1:3,7:9);
psi=eta(3);
R_T = [cos(psi) -sin(psi) 0;
       sin(psi) cos(psi) 0;
       0 0 1]';
eta_tilde = eta_hat - eta;
nu_tilde = nu_hat - nu;

z2_nu_tilde = [z2(1) z2(2)]';
z2_r_tilde = z2(3);

delta_nu_tilde = 0.8;
delta_r_tilde = 1;

K2_func = Gamma2*[ 1/sqrt(z2_nu_tilde'*z2_nu_tilde+delta_nu_tilde^2) 0 0;
    0 1/sqrt(z2_nu_tilde'*z2_nu_tilde+delta_nu_tilde^2) 0;
    0 0 1/sqrt(z2_r_tilde^2+delta_r_tilde^2)];


%adapt gains
gamma_ro_delta=40;
gamma_sigma_delta=40;
gamma_w_delta = 200; 
L1 = eye(3)*100;%*2*K1;
L2 = eye(3)*100;%*2*K2;



%%adaptation laws
ro_delta_hat_dot = -gamma_ro_delta*nu_tilde'*tau;
sigma_delta_hat_dot = gamma_sigma_delta*nu_tilde'*D*nu;
w_delta_hat_dot=-gamma_w_delta*R_T'*nu_tilde;

%%State predictor dynamics
eta_hat_dot = -L1*eta_tilde + R_T'*nu;
nu_hat_dot = -L2*nu_tilde + M\(ro_delta_hat*tau+R_T*w_delta_hat-C*nu-sigma_delta_hat*D*nu);

%debug
% sigma_delta_hat =1;
% ro_delta_hat = 1;
% w_delta_hat = [0 0 0]';
tau =(-R_T*w_delta_hat + M*alpha_dot + C*nu + sigma_delta_hat*D*nu - K2_func*z2)/ro_delta_hat;
%tau = M*alpha_dot + C*nu- K2_func*z2;

== matlab function Adaptive_control_CSAD_model/L1 Cascade/CSAD parameters ==
  data: model output; Nu input
function model = fcn(Nu)

X_u		= -5.35;		
X_uu 	=  0;		
X_uuu	= -19.6312;

Y_v		= -10.16;   
Y_vv	= -0.8647;
Y_vvv	= -681.1745;	

Y_r		= -7.25;
Y_rr	= -3.45;
Y_rrr   = 0;

N_v		= 0;		
N_vv	= -0.2088;
N_vvv = 0;

N_r		= -14.55;
N_rr	= -9.9597;
N_rrr	= -0.3101;

N_rv	= 0.08;	
N_vr	= 0.08;
Y_rv	= -0.805;			
Y_vr	= -0.845;

X_ud =     -10;
Y_vd =     -105;
Y_rd =     -0.525;
N_vd =     -0.157;	
N_rd =     -3.4950;

Nur  = -Y_rd;
Nuv  = -(Y_vd-X_ud);
Yur  = -X_ud;

x_g     = 0.0375;
m       = 127.92;
I_z     = 61.967;

u   = Nu(1);
v   = Nu(2);
r   = Nu(3);

d_11 = - X_u - X_uu*abs(u) - X_uuu*u^2;
d_22 = - Y_v - Y_vv*abs(v) - Y_rv*abs(r) - Y_vvv*v^2;
d_23 = - Y_r - Y_rr*abs(r) - Y_vr*abs(v) - Y_rrr*r^2 - Yur*u;
d_32 = - N_v - N_vv*abs(v) - N_rv*abs(r) - N_vvv*v^2 - Nuv*u;
d_33 = - N_r - N_rr*abs(r) - N_vr*abs(v) - N_rrr*r^2 - Nur*u;

D    = [d_11  0     0
        0     d_22  d_23
        0     d_32  d_33];

CA=[0                            0          Y_vd*v+Y_rd*r;
    0                            0                -X_ud*u;
    -Y_rd*r-Y_vd*v               X_ud*u                0];

CRB=[0             0     -m*(x_g*r+v);
     0             0      m*u;
     m*(x_g*r+v) -m*u     0]; 

C=CRB+CA;

M_RB_c=[m     0      0;
        0     m      m*x_g;
        0     m*x_g  I_z];

M_A_c=[-X_ud    0      0;
         0    -Y_vd  -Y_rd;
         0    -N_vd  -N_rd];     
    
M = M_RB_c + M_A_c;

model=[M C D];

== matlab function Adaptive_control_CSAD_model/fourcorner tracking1 ==
  data: t input; Eta_t output; Eta_t_dot output; Eta_t_ddot output; eta input
function [ Eta_t, Eta_t_dot, Eta_t_ddot]   =  fourcorner_tracking(t,eta)

v_t = 0.15;

etaP = [5 7 7 7 5 5;
       -1 -1 1 1 1 -1;
        0 0 0 pi/4 pi/4 0];
Eta_t_dot = [0;0;0];
Eta_t_ddot = [0;0;0];

Eta_t = [5;-1;0];
persistent point ;
if(isempty(point))
    Eta_t = [5;-1;0];
    point = 1;
    
    
end



switch point
    case 1
        Eta_t = etaP(:,2);
         if ((abs((Eta_t(1)- eta(1))) <0.01 ) ==1  ) && ((abs(Eta_t(2)-eta(2))<0.01) ==1) && (abs(Eta_t(3)-rad2deg(eta(3)))<3 == 1)
            point = 2;
            return;
         end
        
        
    case 2
        Eta_t = etaP(:,3);
        if((abs((Eta_t(1)- eta(1))) <0.01 ) ==1  ) && ((abs(Eta_t(2)-eta(2))<0.01) ==1) && (abs(Eta_t(3)-rad2deg(eta(3)))<3 == 1) 
            point = 3;
            return;
         end
    case 3
        Eta_t = etaP(:,4);
        if((abs((Eta_t(1)- eta(1))) <0.01 ) ==1  ) && ((abs(Eta_t(2)-eta(2))<0.01) ==1) && (rad2deg(abs(Eta_t(3)-eta(3)))<3 == 1)  
            point = 4;
            return;
            
         end
    case 4
        Eta_t = etaP(:,5);
        if((abs((Eta_t(1)- eta(1))) <0.01 ) ==1  ) && ((abs(Eta_t(2)-eta(2))<0.01) ==1) && (rad2deg(abs(Eta_t(3)-eta(3)))<3 == 1) 
            point = 5; 
            return;
         end
    case 5
        Eta_t = etaP(:,6);
        if((abs((Eta_t(1)- eta(1))) <0.01 ) ==1  ) && ((abs(Eta_t(2)-eta(2))<0.01) ==1) && (abs(Eta_t(3)-rad2deg(eta(3)))<3 == 1) 
            point = 6;
            
            return;
         end

    otherwise
        

end
end
%(abs(Eta_t(2)-eta(2))<0.01) &&
